simulink model "verify_coeff_simulink"  (R2022b)
settings: Solver=VariableStepAuto  StartTime=0.0  StopTime=10.0  RelTol=1e-3
libraries: aerolibtransform2 x1
settings Model: Creator=Komsun  LastModifiedBy=Komsun

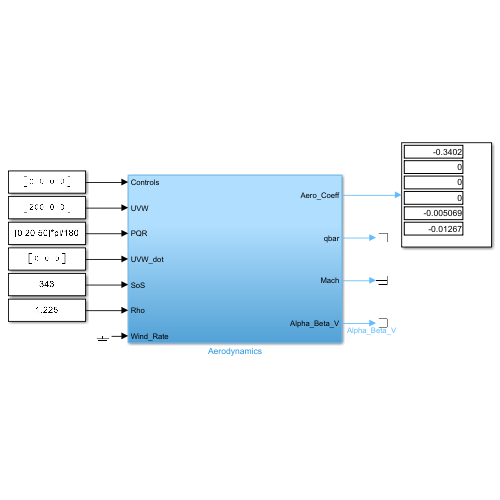
[thumbnail: Simulink's stored preview of the top-level diagram]
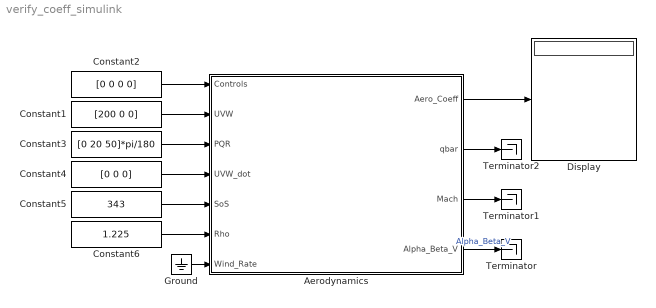
== system verify_coeff_simulink ==
  Aerodynamics : Subsystem
  Constant1 : Constant  Value=[200 0 0]
  Constant2 : Constant  Value=[0 0 0 0]
  Constant3 : Constant  Value=[0 20 50]*pi/180
  Constant4 : Constant  Value=[0 0 0]
  Constant5 : Constant  Value=343
  Constant6 : Constant  Value=1.225
  Display : Display
  Ground : Ground
  Terminator : Terminator
  Terminator1 : Terminator
  Terminator2 : Terminator
  wires:
  Aerodynamics/4(Alpha_Beta_V) -> Terminator/1  "Alpha_Beta_V"
  Aerodynamics/3(Mach) -> Terminator1/1
  Aerodynamics/2(qbar) -> Terminator2/1
  Aerodynamics/1(Aero_Coeff) -> Display/1
  Constant1/1 -> Aerodynamics/2(UVW)
  Constant2/1 -> Aerodynamics/1(Controls)
  Constant3/1 -> Aerodynamics/3(PQR)
  Constant4/1 -> Aerodynamics/4("UVW_dot ")
  Constant5/1 -> Aerodynamics/5(SoS)
  Constant6/1 -> Aerodynamics/6(Rho)
  Ground/1 -> Aerodynamics/7(Wind_Rate)

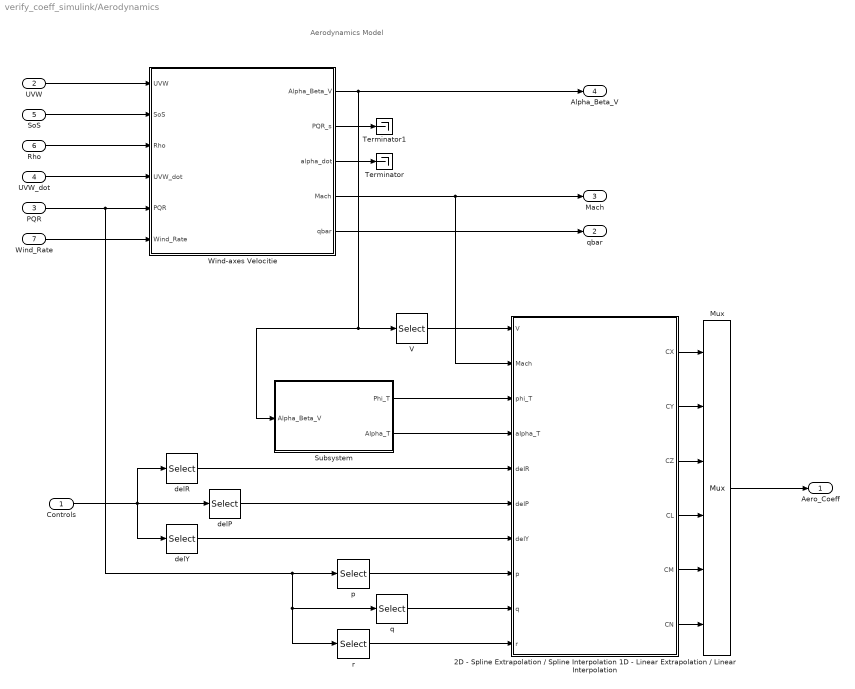
== system verify_coeff_simulink/Aerodynamics ==
  note: Aerodynamics Model
  Controls : Inport
  UVW : Inport  Port=2
  PQR : Inport  Port=3
  "UVW_dot " : Inport  Port=4
  SoS : Inport  Port=5
  Rho : Inport  Port=6
  Wind_Rate : Inport  Port=7
  2D - Spline Extrapolation / Spline Interpolation 1D - Linear Extrapolation / Linear Interpolation : MATLAB Function  TreatAsAtomicUnit=on
  Mux : Mux  Inputs=6
  Subsystem : Subsystem
  Terminator : Terminator
  Terminator1 : Terminator
  V : Selector  InputPortWidth=3  IndexOptions=Index vector (dialog)  Indices=[3]  OutputSizes=1
  Wind-axes Velocitie : Subsystem
  delP : Selector  InputPortWidth=4  IndexOptions=Index vector (dialog)  Indices=[3]  OutputSizes=1
  delR : Selector  InputPortWidth=4  IndexOptions=Index vector (dialog)  Indices=[2]  OutputSizes=1
  delY : Selector  InputPortWidth=4  IndexOptions=Index vector (dialog)  Indices=[4]  OutputSizes=1
  p : Selector  InputPortWidth=3  IndexOptions=Index vector (dialog)  Indices=[1]  OutputSizes=1
  q : Selector  InputPortWidth=3  IndexOptions=Index vector (dialog)  Indices=[2]  OutputSizes=1
  r : Selector  InputPortWidth=3  IndexOptions=Index vector (dialog)  Indices=[3]  OutputSizes=1
  Aero_Coeff : Outport
  qbar : Outport  Port=2
  Mach : Outport  Port=3
  Alpha_Beta_V : Outport  Port=4
  wires:
  Wind-axes Velocitie/1(Alpha_Beta_V) -> Subsystem/1(Alpha_Beta_V), V/1, Alpha_Beta_V/1
  UVW/1 -> Wind-axes Velocitie/1(UVW)
  Mux/1 -> Aero_Coeff/1
  Wind-axes Velocitie/4(Mach) -> 2D - Spline Extrapolation / Spline Interpolation 1D - Linear Extrapolation / Linear Interpolation/2(Mach), Mach/1
  Wind-axes Velocitie/5(qbar) -> qbar/1
  SoS/1 -> Wind-axes Velocitie/2(SoS)
  Rho/1 -> Wind-axes Velocitie/3(Rho)
  "UVW_dot "/1 -> Wind-axes Velocitie/4(UVW_dot)
  PQR/1 -> r/1, q/1, p/1, Wind-axes Velocitie/5(PQR)
  Wind_Rate/1 -> Wind-axes Velocitie/6(Wind_Rate)
  Wind-axes Velocitie/3(alpha_dot) -> Terminator/1
  Wind-axes Velocitie/2(PQR_s) -> Terminator1/1
  Subsystem/2(Alpha_T) -> 2D - Spline Extrapolation / Spline Interpolation 1D - Linear Extrapolation / Linear Interpolation/4(alpha_T)
  V/1 -> 2D - Spline Extrapolation / Spline Interpolation 1D - Linear Extrapolation / Linear Interpolation/1(V)
  Subsystem/1(Phi_T) -> 2D - Spline Extrapolation / Spline Interpolation 1D - Linear Extrapolation / Linear Interpolation/3(phi_T)
  Controls/1 -> delY/1, delR/1, delP/1
  delR/1 -> 2D - Spline Extrapolation / Spline Interpolation 1D - Linear Extrapolation / Linear Interpolation/5(delR)
  delP/1 -> 2D - Spline Extrapolation / Spline Interpolation 1D - Linear Extrapolation / Linear Interpolation/6(delP)
  delY/1 -> 2D - Spline Extrapolation / Spline Interpolation 1D - Linear Extrapolation / Linear Interpolation/7(delY)
  p/1 -> 2D - Spline Extrapolation / Spline Interpolation 1D - Linear Extrapolation / Linear Interpolation/8(p)
  q/1 -> 2D - Spline Extrapolation / Spline Interpolation 1D - Linear Extrapolation / Linear Interpolation/9(q)
  r/1 -> 2D - Spline Extrapolation / Spline Interpolation 1D - Linear Extrapolation / Linear Interpolation/10(r)
  2D - Spline Extrapolation / Spline Interpolation 1D - Linear Extrapolation / Linear Interpolation/1(CX) -> Mux/1
  2D - Spline Extrapolation / Spline Interpolation 1D - Linear Extrapolation / Linear Interpolation/2(CY) -> Mux/2
  2D - Spline Extrapolation / Spline Interpolation 1D - Linear Extrapolation / Linear Interpolation/3(CZ) -> Mux/3
  2D - Spline Extrapolation / Spline Interpolation 1D - Linear Extrapolation / Linear Interpolation/4(CL) -> Mux/4
  2D - Spline Extrapolation / Spline Interpolation 1D - Linear Extrapolation / Linear Interpolation/5(CM) -> Mux/5
  2D - Spline Extrapolation / Spline Interpolation 1D - Linear Extrapolation / Linear Interpolation/6(CN) -> Mux/6

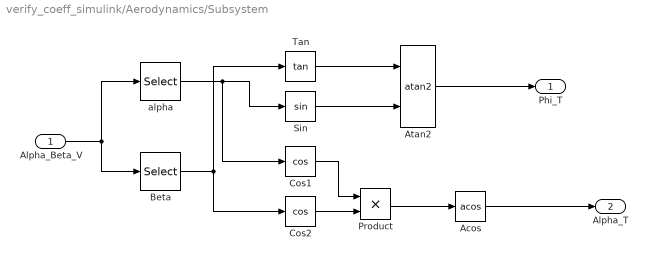
== system verify_coeff_simulink/Aerodynamics/Subsystem ==
  Alpha_Beta_V : Inport
  Acos : Trigonometry  Operator=acos
  Atan2 : Trigonometry  Operator=atan2
  Beta : Selector  InputPortWidth=3  IndexOptions=Index vector (dialog)  Indices=[2]  OutputSizes=1
  Cos1 : Trigonometry  Operator=cos
  Cos2 : Trigonometry  Operator=cos
  Product : Product
  Sin : Trigonometry
  Tan : Trigonometry  Operator=tan
  alpha : Selector  InputPortWidth=3  IndexOptions=Index vector (dialog)  Indices=[1]  OutputSizes=1
  Phi_T : Outport
  Alpha_T : Outport  Port=2
  wires:
  Alpha_Beta_V/1 -> alpha/1, Beta/1
  Beta/1 -> Tan/1, Cos2/1
  Tan/1 -> Atan2/1
  Sin/1 -> Atan2/2
  Atan2/1 -> Phi_T/1
  alpha/1 -> Cos1/1, Sin/1
  Cos1/1 -> Product/1
  Cos2/1 -> Product/2
  Product/1 -> Acos/1
  Acos/1 -> Alpha_T/1

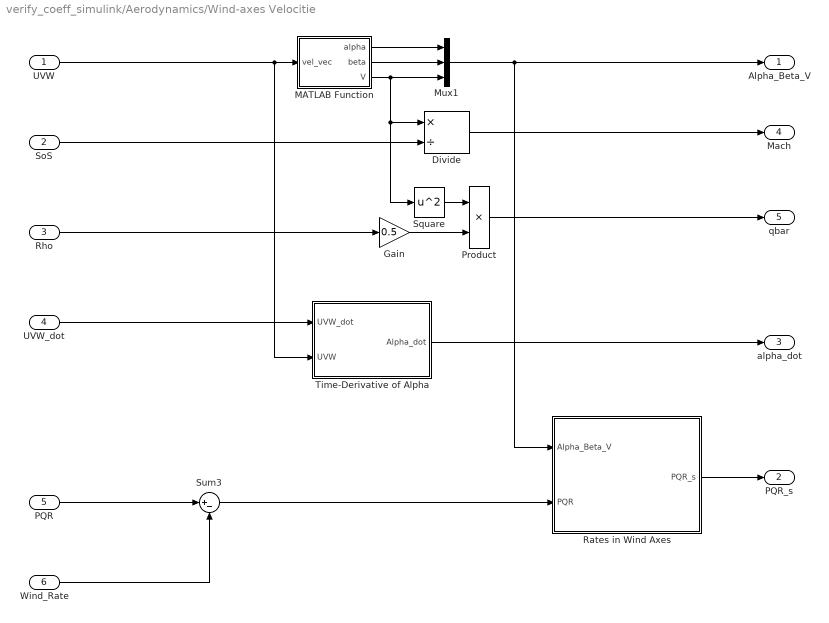
== system verify_coeff_simulink/Aerodynamics/Wind-axes Velocitie ==
  UVW : Inport
  SoS : Inport  Port=2
  Rho : Inport  Port=3
  UVW_dot : Inport  Port=4
  PQR : Inport  Port=5
  Wind_Rate : Inport  Port=6
  Divide : Product  Inputs=*/
  Gain : Gain  Gain=0.5
  MATLAB Function : MATLAB Function  TreatAsAtomicUnit=on
  Mux1 : Mux  Inputs=3
  Product : Product
  Rates in Wind Axes : Subsystem
  Square : Math  Operator=square
  Sum3 : Sum  Inputs=|+-  InputSameDT=on  SaturateOnIntegerOverflow=on  OutDataTypeStr=Inherit: Same as first input
  Time-Derivative of Alpha : Subsystem
  Alpha_Beta_V : Outport
  PQR_s : Outport  Port=2
  alpha_dot : Outport  Port=3
  Mach : Outport  Port=4
  qbar : Outport  Port=5
  wires:
  UVW_dot/1 -> Time-Derivative of Alpha/1(UVW_dot)
  Time-Derivative of Alpha/1(Alpha_dot) -> alpha_dot/1
  Product/1 -> qbar/1
  Rho/1 -> Gain/1
  SoS/1 -> Divide/2
  Divide/1 -> Mach/1
  Mux1/1 -> Rates in Wind Axes/1(Alpha_Beta_V), Alpha_Beta_V/1
  UVW/1 -> Time-Derivative of Alpha/2(UVW), MATLAB Function/1(vel_vec)
  MATLAB Function/1(alpha) -> Mux1/1
  MATLAB Function/2(beta) -> Mux1/2
  MATLAB Function/3(V) -> Square/1, Divide/1, Mux1/3
  Rates in Wind Axes/1(PQR_s) -> PQR_s/1
  Sum3/1 -> Rates in Wind Axes/2(PQR)
  PQR/1 -> Sum3/1
  Wind_Rate/1 -> Sum3/2
  Square/1 -> Product/1
  Gain/1 -> Product/2

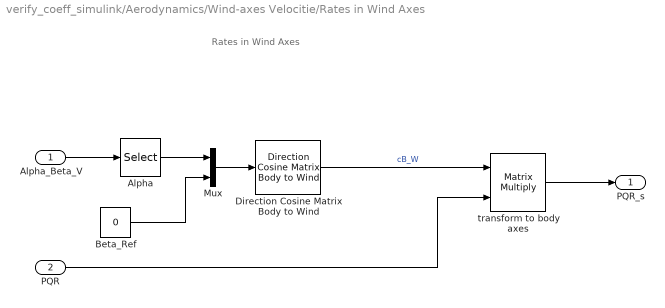
== system verify_coeff_simulink/Aerodynamics/Wind-axes Velocitie/Rates in Wind Axes ==
  note: Rates in Wind Axes
  Alpha_Beta_V : Inport
  PQR : Inport  Port=2
  Alpha : Selector  InputPortWidth=3  IndexOptions=Index vector (dialog)  Indices=[1]  OutputSizes=1
  Beta_Ref : Constant  Value=0
  Direction Cosine Matrix Body to Wind : aerolibtransform2/Direction Cosine Matrix Body to Wind
  Mux : Mux  Inputs=2
  transform to body axes : Product  Inputs=**  Multiplication=Matrix(*)  InputSameDT=on  SaturateOnIntegerOverflow=on  OutDataTypeStr=Inherit: Same as first input
  PQR_s : Outport
  wires:
  Alpha_Beta_V/1 -> Alpha/1
  Alpha/1 -> Mux/1
  Direction Cosine Matrix Body to Wind/1 -> transform to body axes/1  "cB_W"
  PQR/1 -> transform to body axes/2
  transform to body axes/1 -> PQR_s/1
  Mux/1 -> Direction Cosine Matrix Body to Wind/1
  Beta_Ref/1 -> Mux/2

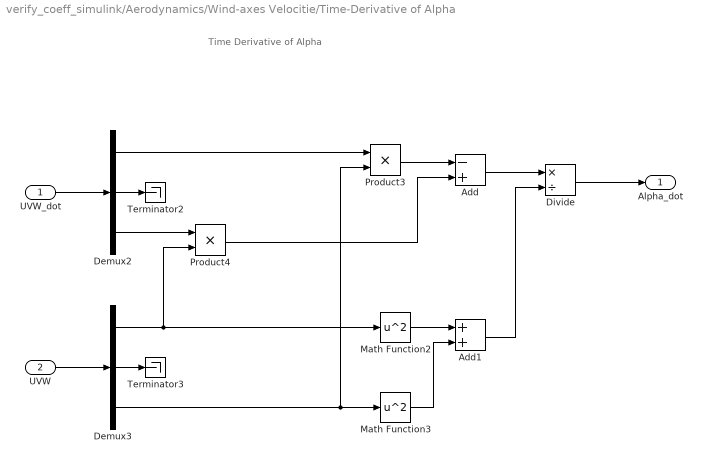
== system verify_coeff_simulink/Aerodynamics/Wind-axes Velocitie/Time-Derivative of Alpha ==
  note: Time Derivative of Alpha
  UVW_dot : Inport
  UVW : Inport  Port=2
  Add : Sum  Inputs=-+
  Add1 : Sum
  Demux2 : Demux  Outputs=3
  Demux3 : Demux  Outputs=3
  Divide : Product  Inputs=*/
  Math Function2 : Math  Operator=square  SignedPower=on
  Math Function3 : Math  Operator=square  SignedPower=on
  Product3 : Product
  Product4 : Product
  Terminator2 : Terminator
  Terminator3 : Terminator
  Alpha_dot : Outport
  wires:
  UVW_dot/1 -> Demux2/1
  Demux2/2 -> Terminator2/1
  Demux2/1 -> Product3/1
  UVW/1 -> Demux3/1
  Demux3/2 -> Terminator3/1
  Demux3/3 -> Math Function3/1, Product3/2
  Demux2/3 -> Product4/1
  Demux3/1 -> Math Function2/1, Product4/2
  Product4/1 -> Add/2
  Product3/1 -> Add/1
  Add/1 -> Divide/1
  Math Function2/1 -> Add1/1
  Math Function3/1 -> Add1/2
  Add1/1 -> Divide/2
  Divide/1 -> Alpha_dot/1

== matlab function verify_coeff_simulink/Aerodynamics/Wind-axes Velocitie/MATLAB Function ==
  data: vel_vec input; alpha output; beta output; V output
function [alpha, beta, V] = calc_abv(vel_vec)

u = vel_vec(1);
v = vel_vec(2);
w = vel_vec(3);

V = norm([u v w]);          % [m/s] UAV total Speed
alpha = atan2(w,u);          % [rad] angle of attack
beta  = asin(v/V);          % [rad] sideslip angles

end

== matlab function verify_coeff_simulink/Aerodynamics/2D - Spline Extrapolation // Spline Interpolation 1D - Linear Extrapolation // Linear Interpolation ==
  data: V input; Mach input; CX output; phi_T input; alpha_T input; delR input; delP input; delY input; CY output; CZ output; CL output; CM output; CN output; p input; q input; r input
function [CX, CY, CZ, CL, CM, CN] = AeroCoef(V, Mach,phi_T, alpha_T, delR, delP, delY, p, q, r)

dat = load('UAV_Data.mat');
dat.Tbl_ALPHAT = dat.Tbl_ALPHAT;    % convert to rad
% alpha_T = alpha_T *180/pi;            % convert to degree

del_eff = (abs(delP) + abs(delY))/2;


B2A = rot1(-phi_T);                            % Body-to-Aeroballistics

delARPY = B2A *[delR; delP; delY];
delR_A = delARPY(1);
delP_A = delARPY(2);
delY_A = delARPY(3);

pqrA = B2A * [p; q; r];
pA = pqrA(1);
qA = pqrA(2);
rA = pqrA(3);

method = 'linear'; % 'spline', 'nearest'
method2 = 'spline';

CX_a = interp1(dat.Tbl_MACH, dat.Tbl_CX_0, Mach, method,'extrap') + interp1(dat.Tbl_MACH, dat.Tbl_CX_ALPHAT, Mach, method,'extrap')*alpha_T...
     + interp1(dat.Tbl_MACH, dat.Tbl_CX_DEL_EFF, Mach, method,'extrap')*(del_eff)^2;

CY_a = interp2(dat.Tbl_ALPHAT, dat.Tbl_MACH, dat.Tbl_CY_PHIT, alpha_T*180/pi, Mach, method2)*sin(4*phi_T)...
     + interp1(dat.Tbl_MACH, dat.Tbl_CY_DEL_Y, Mach, method,'extrap')*delY_A;

CZ_a = interp2(dat.Tbl_ALPHAT, dat.Tbl_MACH, dat.Tbl_CZ_0, alpha_T*180/pi, Mach, method2)...
     + interp2(dat.Tbl_ALPHAT, dat.Tbl_MACH, dat.Tbl_CZ_PHIT, alpha_T*180/pi, Mach, method2)*(sin(2*phi_T))^2 ...
     + interp1(dat.Tbl_MACH, dat.Tbl_CZ_DEL_P, Mach, method,'extrap')*delP_A;

CL_a = interp1(dat.Tbl_MACH, dat.Tbl_CL_ALPHAT, Mach, method,'extrap')*(alpha_T^2)*sin(4*phi_T) ...
     + interp1(dat.Tbl_MACH, dat.Tbl_CL_P, Mach, method,'extrap')*(dat.D/(2*V))*pA ...
     + interp1(dat.Tbl_MACH, dat.Tbl_CL_DEL_R, Mach, method,'extrap')*delR_A;

CM_a = interp2(dat.Tbl_ALPHAT, dat.Tbl_MACH, dat.Tbl_CM_0, alpha_T*180/pi, Mach, method2) ...
     + interp2(dat.Tbl_ALPHAT, dat.Tbl_MACH, dat.Tbl_CM_PHIT, alpha_T*180/pi, Mach, method2)*(sin(2*phi_T))^2 ...
     + interp1(dat.Tbl_MACH, dat.Tbl_CM_Q, Mach, method,'extrap')*(dat.D/(2*V))*qA ...
     + interp1(dat.Tbl_MACH, dat.Tbl_CM_DEL_P, Mach, method,'extrap')*delP_A ...
     - CZ_a*(dat.XCG - dat.XREF)/dat.D;

CN_a = interp2(dat.Tbl_ALPHAT, dat.Tbl_MACH, dat.Tbl_CN_PHIT, alpha_T*180/pi, Mach, method2)*sin(4*phi_T)...
     + interp1(dat.Tbl_MACH, dat.Tbl_CN_R, Mach, method,'extrap')*(dat.D/(2*V))*rA ...
     + interp1(dat.Tbl_MACH, dat.Tbl_CN_DEL_Y, Mach, method,'extrap')*delY_A ...
     + CY_a*(dat.XCG - dat.XREF)/dat.D;

%% Aerodynamics Coefficients in body coordinate
CXYZ = B2A.' * [CX_a; CY_a; CZ_a];
CX = CXYZ(1);
CY = CXYZ(2);
CZ = CXYZ(3);

CLMN = B2A.' * [CL_a; CM_a; CN_a];
CL = CLMN(1);
CM = CLMN(2);
CN = CLMN(3);

function out = rot1(x)
    out = [1 0 0; 0 cos(x) sin(x); 0 -sin(x) cos(x)];
end

end
